simulink model "KoopmanMPC"  (R2023b)
settings: Solver=FixedStepAuto  StartTime=0.0  StopTime=inf  FixedStep=0.01  RelTol=1e-3
values from neighbouring files (symbols this model uses):
  ref_resampled_4 = [-0.0434326850921 1.00739834805 -5.2965480502 -0.0275886266971 -0.00523965410955 0.0242941259565 0.000763390489614 -0.0605545134458 1.09554308151 -5.3213592223 -0.0277571536527 -0.0053597164637 ... (2807 elements, 7x401)]    [circle_resampled_trajectory_4.mat]
undefined symbols (not defined in the file or in its folder): canChannel
libraries: canmsglib x15, canlib x11, simulink x11, dspfdesign x7, auroraNDILibrary x1
(part 1 of 2)
settings Model: Creator=86188  LastModifiedBy=86188
settings SolverCC: ConcurrentTasks=on  PositivePriorityOrder=on
settings OptimizationCC: BlockReduction=off  OptimizeBlockIOStorage=off  BufferReuse=off
settings DebuggingCC: AlgebraicLoopMsg=none  TasksWithSamePriorityMsg=none
settings HardwareCC: ProdBitPerLong=64  ProdLongLongMode=on  ProdHWDeviceType=Intel->x86-64 (Linux 64)
settings RTWCC: Description=Simulink Real-Time  SystemTargetFile=slrealtime.tlc  TemplateMakefile=slrealtime_default_tmf  Toolchain=Simulink Real-Time Toolchain  BuildConfiguration=Faster Runs  CodeExecutionProfiling=on  TargetLang=C++

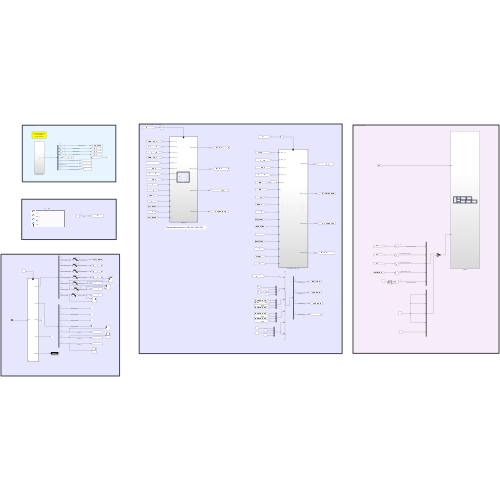
[thumbnail: Simulink's stored preview of the top-level diagram]
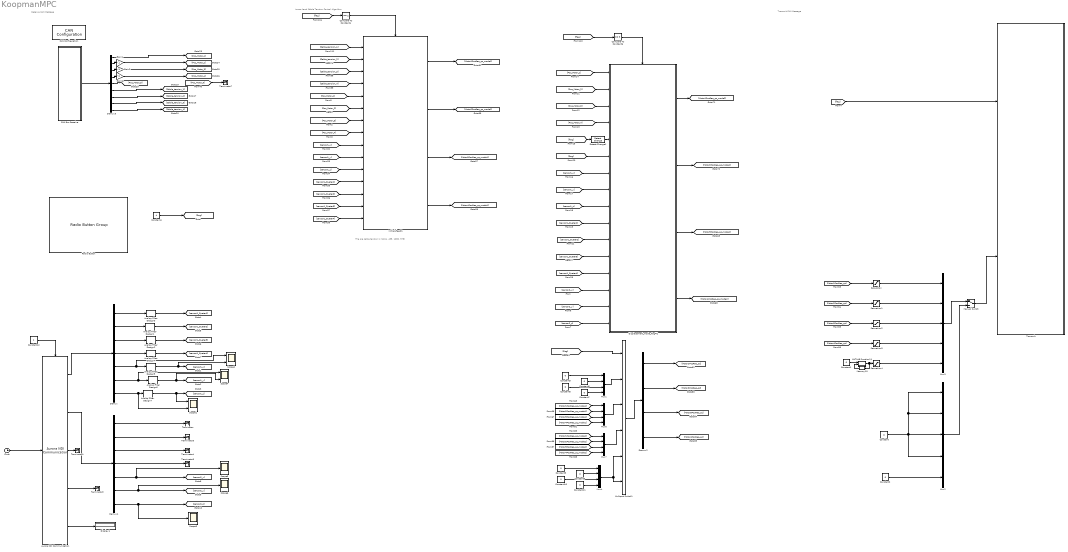
== system KoopmanMPC ==
  note: Transmit CAN Message
  note: Lower level Cable Tension Control Algorithm
  note: The pre cable tension is (1104, 455, 1080, 978)
  note: Receive CAN Message
  Analog Filter Design{1..5} (5 alike) : dspfdesign/Analog Filter Design  method=Butterworth  filttype=Lowpass  N=2  Wlo=4  Whi=80  Rp=2  Rs=40
  Analog Filter Design6 : dspfdesign/Analog Filter Design  method=Butterworth  filttype=Lowpass  N=1  Wlo=4  Whi=80  Rp=2  Rs=40
  Analog Filter Design7 : dspfdesign/Analog Filter Design  method=Butterworth  filttype=Lowpass  N=1  Wlo=4  Whi=80  Rp=2  Rs=40
  Aurora NDI Communication : auroraNDILibrary/Aurora NDI Communication  SampleFrequency=40  comNumber=4
  CAN Bus Receive : Subsystem
  CAN Configuration : canlib/CAN Configuration  BlockHandle=7005.0032  Device=PEAK-System PCAN-USB (PCAN_USBBUS1)  DeviceMenu=PEAK-System PCAN-USB (PCAN_USBBUS1)  ObjConstructor=canChannel('PEAK-System', 'PCAN_USBBUS1')  BusSpeed=500000  EnableBitParameters=off  AckMode=Normal
  Clock : Clock
  Compare To Constant4 : simulink/Logic and Bit Operations/Compare To Constant  relop===  const=2  OutDataTypeStr=boolean
  Compare To Constant6 : simulink/Logic and Bit Operations/Compare To Constant  relop===  const=3  OutDataTypeStr=boolean
  Constant{,1..3,5..11} (11 alike) : Constant  Value=0
  Constant12 : Constant
  Constant4 : Constant  Value=4
  Demux : Demux  Outputs=7
  Demux1 : Demux  Outputs=7
  Demux2 : Demux
  Demux3 : Demux  Outputs=9
  Detect Change1 : simulink/Logic and Bit Operations/Detect Change  vinit=0  OutDataTypeStr=boolean
  Displacement_mode_flag=2 : Subsystem
  Display1 : Display
  Gain1 : Gain  Gain=-1
  Gain2 : Gain  Gain=-1
  Gain6 : Gain  Gain=-1
  Initial_flag=1 : Subsystem
  MATLAB Function11 : MATLAB Function  TreatAsAtomicUnit=on
  Manual Switch : ManualSwitch
  Memory10 : Memory
  Multiport Switch1 : MultiPortSwitch  Inputs=4  DataPortForDefault=Additional data port  SaturateOnIntegerOverflow=off  InputSameDT=off
  Mux{1,4,6..7} (4 alike) : Mux
  Mux2 : Mux  Inputs=5
  Mux3 : Mux  Inputs=5
  Radio Button : RadioButtonGroup  SelectedLabel=End  ButtonGroupName=Group
      settings: Values={{'Initial', 'PreTension', 'MPC', 'End'}, [1 2 3 4]}
  Saturation{,1..3} (4 alike) : Saturate  UpperLimit=6000  LowerLimit=-6000
  Saturation4 : Saturate  UpperLimit=80  LowerLimit=-80
  Scope1 : Scope  NumInputPorts=2
  Scope2 : Scope  NumInputPorts=2
  Scope3 : Scope
  Scope4 : Scope  NumInputPorts=2
  Scope5 : Scope
  Scope6 : Scope
  Terminator{,1..5,7} (7 alike) : Terminator
  Transmit : Subsystem
  wires:
  Multiport Switch1/1 -> Demux2/1
  [Motor1PosReq_qc_mode2] -> Mux7/1
  Manual Switch/1 -> Transmit/2(Input)
  [Motor3PosReq_qc_mode2] -> Mux7/3
  [Motor2PosReq_qc_mode1] -> Mux6/2
  [Motor4PosReq_qc_mode1] -> Mux6/4
  Initial_flag=1/2(Motor2_pos_req_qc) -> [Motor2PosReq_qc_mode1]
  Initial_flag=1/3(Motor3PosReq_qc) -> [Motor3PosReq_qc_mode1]
  [flag] -> Compare To Constant4/1
  Displacement_mode_flag=2/3(Motor3PosReq_qc) -> [Motor3PosReq_qc_mode2]
  Displacement_mode_flag=2/2(Motor2_pos_req_qc) -> [Motor2PosReq_qc_mode2]
  Displacement_mode_flag=2/4(Motor4PosReq_qc) -> [Motor4PosReq_qc_mode2]
  [Motor3PosReq_qc] -> Saturation2/1
  [flag] -> Transmit/1(flag)
  [Motor1PosReq_qc_mode1] -> Mux6/1
  Displacement_mode_flag=2/1(Motor1PosReq_qc) -> [Motor1PosReq_qc_mode2]
  Initial_flag=1/4(Motor4PosReq_qc) -> [Motor4PosReq_qc_mode1]
  [Cable_tension_4] -> Initial_flag=1/4(Force_sensor_4_g)
  Compare To Constant4/1 -> Initial_flag=1/Enable
  [flag] -> Compare To Constant6/1
  [Cable_tension_3] -> Initial_flag=1/3(Force_sensor_3_g)
  [Motor3PosReq_qc_mode1] -> Mux6/3
  Mux2/1 -> Manual Switch/2
  [Motor4PosReq_qc_mode2] -> Mux7/4
  [Motor2PosReq_qc_mode2] -> Mux7/2
  Compare To Constant6/1 -> Displacement_mode_flag=2/Enable
  [Cable_tension_2] -> Initial_flag=1/2(Force_sensor_2_g)
  [Cable_tension_1] -> Initial_flag=1/1(Force_sensor_1_g)
  Initial_flag=1/1(Motor1PosReq_qc) -> [Motor1PosReq_qc_mode1]
  [Pos_Motor_2] -> Displacement_mode_flag=2/2(Pos_Motor_2_qc)
  [Pos_Motor_1] -> Displacement_mode_flag=2/1(Pos_Motor_1_qc)
  [Pos_Motor_3] -> Displacement_mode_flag=2/3(Pos_Motor_3_qc)
  [Pos_Motor_4] -> Displacement_mode_flag=2/4(Pos_Motor_4_qc)
  [flag] -> Detect Change1/1
  [flag] -> Displacement_mode_flag=2/6(flag)
  Detect Change1/1 -> Displacement_mode_flag=2/5(flag_change)
  Saturation4/1 -> Mux3/5  "Motor5PosReq_qc_final"
  Mux3/1 -> Manual Switch/1
  Saturation3/1 -> Mux3/4  "Motor4PosReq_qc_final"
  Saturation/1 -> Mux3/1  "Motor1PosReq_qc_final"
  Saturation1/1 -> Mux3/2  "Motor2PosReq_qc_final"
  Saturation2/1 -> Mux3/3  "Motor3PosReq_qc_final"
  [Motor2PosReq_qc] -> Saturation1/1
  [Motor4PosReq_qc] -> Saturation3/1
  MATLAB Function11/1(y) -> Memory10/1, Saturation4/1
  Memory10/1 -> MATLAB Function11/2(u_last)
  Demux2/1 -> [Motor1PosReq_qc]  "Motor1PosReq_qc"
  Demux2/2 -> [Motor2PosReq_qc]  "Motor2PosReq_qc"
  Demux2/3 -> [Motor3PosReq_qc]  "Motor3PosReq_qc"
  Demux2/4 -> [Motor4PosReq_qc]  "Motor4PosReq_qc"
  Constant1/1 -> MATLAB Function11/1(u)
  Constant/1 -> Mux2/4, Mux2/1, Mux2/2, Mux2/3
  Constant2/1 -> Mux2/5
  [Pos_Motor_1] -> Initial_flag=1/5(Pos_Motor_1_qc)
  [Pos_Motor_2] -> Initial_flag=1/6(Pos_Motor_2_qc)
  [Pos_Motor_3] -> Initial_flag=1/7(Pos_Motor_3_qc)
  [Pos_Motor_4] -> Initial_flag=1/8(Pos_Motor_4_qc)
  [flag] -> Multiport Switch1/1
  [Motor1PosReq_qc] -> Saturation/1
  [sensor1_Quater1] -> Displacement_mode_flag=2/10(q0)
  [sensor1_z] -> Displacement_mode_flag=2/9(z)
  [sensor1_Quater2] -> Displacement_mode_flag=2/11(q1)
  [sensor1_y] -> Displacement_mode_flag=2/8(y)
  [sensor1_Quater3] -> Displacement_mode_flag=2/12(q2)
  [sensor1_x] -> Displacement_mode_flag=2/7(x)
  [sensor1_Quater4] -> Displacement_mode_flag=2/13(q3)
  [sensor1_x] -> Initial_flag=1/9(x)
  [sensor1_y] -> Initial_flag=1/10(y)
  [sensor1_z] -> Initial_flag=1/11(z)
  [sensor1_Quater1] -> Initial_flag=1/12(q0)
  [sensor1_Quater2] -> Initial_flag=1/13(q1)
  [sensor1_Quater3] -> Initial_flag=1/14(q2)
  [sensor1_Quater4] -> Initial_flag=1/15(q3)
  [Pos_Motor_5] -> Terminator7/1
  Gain1/1 -> [Pos_Motor_2]  "RealPos_Motor_2"
  Demux3/2 -> Gain1/1
  Demux3/4 -> Gain6/1
  Gain6/1 -> [Pos_Motor_4]  "RealPos_Motor_4"
  Demux3/7 -> [Cable_tension_2]  "force_sensor_2_org"
  Gain2/1 -> [Pos_Motor_3]  "RealPos_Motor_3"
  Demux3/8 -> [Cable_tension_3]  "force_sensor_3_org"
  Demux3/5 -> [Pos_Motor_5]
  Demux3/3 -> Gain2/1
  Demux3/1 -> [Pos_Motor_1]  "RealPos_Motor_1"
  Demux3/6 -> [Cable_tension_1]  "force_sensor_1_org"
  CAN Bus Receive/1(Outport) -> Demux3/1
  Demux3/9 -> [Cable_tension_4]  "force_sensor_4_org"
  Mux6/1 -> Multiport Switch1/3
  Mux7/1 -> Multiport Switch1/4
  Constant7/1 -> Mux1/4
  Constant5/1 -> Mux1/2
  Constant6/1 -> Mux1/3
  Mux1/1 -> Multiport Switch1/2
  Constant3/1 -> Mux1/1
  Constant4/1 -> [flag]  "flag"
  Constant10/1 -> Mux4/3
  Constant9/1 -> Mux4/2
  Constant11/1 -> Mux4/4
  Mux4/1 -> Multiport Switch1/6, Multiport Switch1/5
  Constant8/1 -> Mux4/1
  Demux1/2 -> Terminator3/1  "sensor2_Quater2"
  Demux1/6 -> Scope6/1, [sensor2_y]  "sensor2_y"
  Demux1/4 -> Terminator5/1  "sensor2_Quater4"
  Aurora NDI Communication/2 -> Demux1/1
  Analog Filter Design5/1 -> Scope2/2, [sensor1_x]  "sensor1_x_after"
  Demux1/1 -> Terminator/1  "sensor2_Quater1"
  Aurora NDI Communication/5 -> Display1/1
  Demux/7 -> Analog Filter Design7/1, Scope1/2  "sensor1_z_before"
  Analog Filter Design7/1 -> Scope1/1, [sensor1_z]  "sensor1_z_after"
  Demux1/5 -> [sensor2_x], Scope5/1  "sensor2_x"
  Analog Filter Design6/1 -> Scope4/2, [sensor1_y]  "sensor1_y_after"
  Demux/4 -> Analog Filter Design4/1  "sensor1_Quater4_before"
  Demux1/3 -> Terminator4/1  "sensor2_Quater3"
  Analog Filter Design4/1 -> [sensor1_Quater4]  "sensor1_Quater4_after"
  Demux/5 -> Scope2/1, Analog Filter Design5/1  "sensor1_x_before"
  Analog Filter Design2/1 -> [sensor1_Quater3]  "sensor1_Quater3_after"
  Demux1/7 -> Scope3/1, [sensor2_z]  "sensor2_z"
  Demux/6 -> Analog Filter Design6/1, Scope4/1  "sensor1_y_before"
  Analog Filter Design3/1 -> [sensor1_Quater1]  "sensor1_Quater1_after"
  Demux/1 -> Analog Filter Design3/1  "sensor1_Quater1_before"
  Aurora NDI Communication/1 -> Demux/1
  Demux/2 -> Analog Filter Design1/1  "sensor1_Quater2_before"
  Constant12/1 -> Aurora NDI Communication/Enable
  Aurora NDI Communication/3 -> Terminator1/1
  Clock/1 -> Aurora NDI Communication/1
  Aurora NDI Communication/4 -> Terminator2/1
  Analog Filter Design1/1 -> [sensor1_Quater2]  "sensor1_Quater2_after"
  Demux/3 -> Analog Filter Design2/1  "sensor1_Quater3_before"
  [sensor2_x] -> Displacement_mode_flag=2/14(x1)
  [sensor2_z] -> Displacement_mode_flag=2/16(z1)
  [sensor2_y] -> Displacement_mode_flag=2/15(y1)

== system KoopmanMPC/CAN Bus Receive ==
  CAN Receive : canlib/CAN Receive  BlockHandle=1206.0054  Device=PEAK-System PCAN-USB (PCAN_USBBUS1)  DeviceMenu=PEAK-System PCAN-USB (PCAN_USBBUS1)  ObjConstructor=canChannel('PEAK-System', 'PCAN_USBBUS1')  EnableStandardIDsFilter=off  StdIDsCombo=Allow all  StandardIDs=0  EnableExtendedIDsFilter=off  ExtIDsCombo=Allow all  ExtendedIDs=0  SampleTime=0.01  MsgsPerTimestep=all  InternalFilterUpdateStatus=on  BusOutput=on
  Rate Transition : RateTransition  OutPortSampleTime=0.01
  Subsystem : Subsystem
  Outport : Outport
  wires:
  CAN Receive/1 -> Subsystem/Trigger
  Subsystem/1(Outport1) -> Rate Transition/1
  Rate Transition/1 -> Outport/1
  CAN Receive/2 -> Subsystem/1(In2)

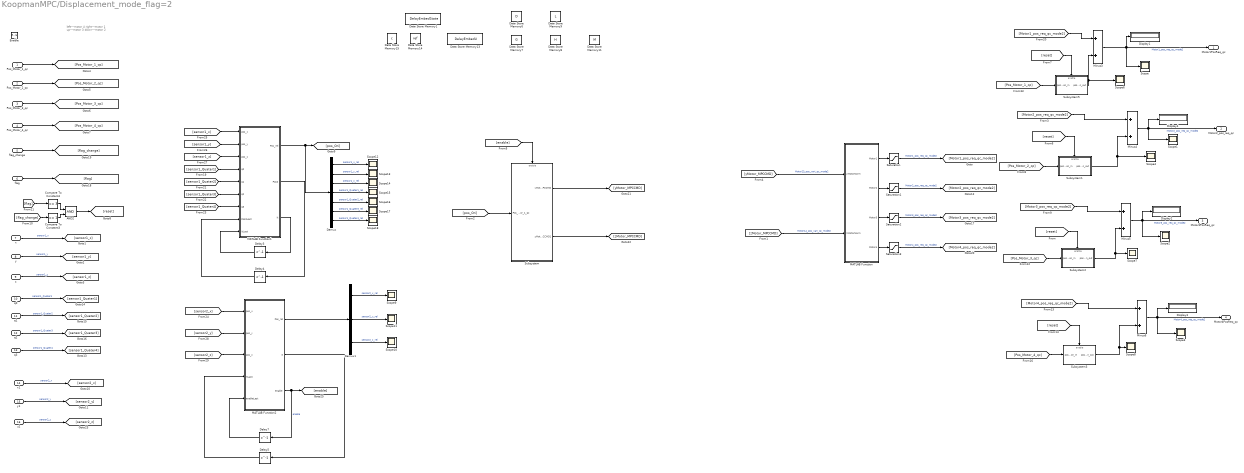
== system KoopmanMPC/Displacement_mode_flag=2 ==
  note: left---motor 4
      | right---motor 1
      | up---motor 3
      | down---motor 2
  Pos_Motor_1_qc : Inport
  Pos_Motor_2_qc : Inport  Port=2
  Pos_Motor_3_qc : Inport  Port=3
  Pos_Motor_4_qc : Inport  Port=4
  flag_change : Inport  Port=5
  flag : Inport  Port=6
  x : Inport  Port=7
  y : Inport  Port=8
  z : Inport  Port=9
  q0 : Inport  Port=10
  q1 : Inport  Port=11
  q2 : Inport  Port=12
  q3 : Inport  Port=13
  x1 : Inport  Port=14
  y1 : Inport  Port=15
  z1 : Inport  Port=16
  Enable : EnablePort  StatesWhenEnabling=reset
  AND2 : Logic  IconShape=distinctive  AllPortsSameDT=off  OutDataTypeStr=boolean
  Compare To Constant3 : simulink/Logic and Bit Operations/Compare To Constant  relop===  const=1  OutDataTypeStr=boolean
  Compare To Constant4 : simulink/Logic and Bit Operations/Compare To Constant  relop===  const=3  OutDataTypeStr=boolean
  Data Store Memory1 : DataStoreMemory  DataStoreName=DelayEmbedState  WriteAfterWriteMsg=warning  InitialValue=zeros(7,2)  ShowAdditionalParam=off  OutDataTypeStr=double
  Data Store Memory11 : DataStoreMemory  DataStoreName=M  WriteAfterWriteMsg=warning  InitialValue=M  ShowAdditionalParam=off  OutDataTypeStr=double
  Data Store Memory13 : DataStoreMemory  DataStoreName=DelayEmbedU  WriteAfterWriteMsg=warning  InitialValue=zeros(2,2)  ShowAdditionalParam=off  OutDataTypeStr=double
  Data Store Memory14 : DataStoreMemory  DataStoreName=ref  WriteAfterWriteMsg=warning  InitialValue=[ref_resampled_4,ref_resampled_4]  ShowAdditionalParam=off  OutDataTypeStr=double
  Data Store Memory15 : DataStoreMemory  DataStoreName=c  WriteAfterWriteMsg=warning  InitialValue=c  ShowAdditionalParam=off  OutDataTypeStr=double
  Data Store Memory6 : DataStoreMemory  DataStoreName=D  WriteAfterWriteMsg=warning  InitialValue=D  ShowAdditionalParam=off  OutDataTypeStr=double
  Data Store Memory7 : DataStoreMemory  DataStoreName=G  WriteAfterWriteMsg=warning  InitialValue=G  ShowAdditionalParam=off  OutDataTypeStr=double
  Data Store Memory8 : DataStoreMemory  DataStoreName=H  WriteAfterWriteMsg=warning  InitialValue=H  ShowAdditionalParam=off  OutDataTypeStr=double
  Data Store Memory9 : DataStoreMemory  DataStoreName=L  WriteAfterWriteMsg=warning  InitialValue=L  ShowAdditionalParam=off  OutDataTypeStr=double
  Delay3 : Delay  DelayLength=1  InitialCondition=1
  Delay4 : Delay  DelayLength=1  InitialCondition=ones(1,7)
  Delay5 : Delay  DelayLength=1  InitialCondition=1
  Delay7 : Delay  DelayLength=1  InitialCondition=0
  Demux : Demux  Outputs=7
  Demux1 : Demux  Outputs=3
  Display{1..4} (4 alike) : Display
  MATLAB Function : MATLAB Function  TreatAsAtomicUnit=on
  MATLAB Function1 : MATLAB Function  TreatAsAtomicUnit=on
  MATLAB Function2 : MATLAB Function  TreatAsAtomicUnit=on
  Minus{3..6} (4 alike) : Sum
  Saturation{,1..3} (4 alike) : Saturate  UpperLimit=1200  LowerLimit=-1200
  Scope{,1..4,6..18} (18 alike) : Scope
  Subsystem : Subsystem
  Subsystem1 : Subsystem
  Subsystem2 : Subsystem
  Subsystem3 : Subsystem
  Subsystem5 : Subsystem
  Motor1PosReq_qc : Outport
  Motor2_pos_req_qc : Outport  Port=2
  Motor3PosReq_qc : Outport  Port=3
  Motor4PosReq_qc : Outport  Port=4
  wires:
  Pos_Motor_4_qc/1 -> [Pos_Motor_4_qc]
  Pos_Motor_3_qc/1 -> [Pos_Motor_3_qc]
  Pos_Motor_2_qc/1 -> [Pos_Motor_2_qc]
  Pos_Motor_1_qc/1 -> [Pos_Motor_1_qc]
  flag/1 -> [flag]
  flag_change/1 -> [flag_change]
  [Pos_Motor_1_qc] -> Subsystem5/1(position_in)
  [reset] -> Subsystem5/Enable
  [Motor1_pos_req_qc_mode2] -> Minus3/1
  Minus3/1 -> Scope/1, Display1/1, Motor1PosReq_qc/1  "Motor1_pos_req_qc_mode2"
  Subsystem5/1(position_out) -> Minus3/2, Scope6/1
  [Motor2_pos_req_qc_mode2] -> Minus4/1
  [reset] -> Subsystem1/Enable
  [Pos_Motor_2_qc] -> Subsystem1/1(position_in)
  Minus4/1 -> Scope1/1, Display4/1, Motor2_pos_req_qc/1  "Motor2_pos_req_qc_mode2"
  Minus5/1 -> Scope2/1, Motor3PosReq_qc/1, Display2/1  "Motor3_pos_req_qc_mode2"
  [reset] -> Subsystem2/Enable
  [Pos_Motor_3_qc] -> Subsystem2/1(position_in)
  [Motor3_pos_req_qc_mode2] -> Minus5/1
  Minus6/1 -> Scope3/1, Motor4PosReq_qc/1, Display3/1  "Motor4_pos_req_qc_mode2"
  [reset] -> Subsystem3/Enable
  [Pos_Motor_4_qc] -> Subsystem3/1(position_in)
  [Motor4_pos_req_qc_mode2] -> Minus6/1
  Compare To Constant4/1 -> AND2/1
  Compare To Constant3/1 -> AND2/2
  [flag_change] -> Compare To Constant3/1
  [flag] -> Compare To Constant4/1
  AND2/1 -> [reset]
  Subsystem2/1(position_out) -> Minus5/2, Scope7/1
  Subsystem3/1(position_out) -> Minus6/2, Scope8/1
  Subsystem1/1(position_out) -> Minus4/2, Scope4/1
  x/1 -> [sensor1_x]  "sensor1_x"
  y/1 -> [sensor1_y]  "sensor1_y"
  z/1 -> [sensor1_z]  "sensor1_z"
  q0/1 -> [sensor1_Quater1]  "sensor1_Quater1"
  q1/1 -> [sensor1_Quater2]  "sensor1_Quater2"
  q3/1 -> [sensor1_Quater4]  "sensor1_Quater4"
  q2/1 -> [sensor1_Quater3]  "sensor1_Quater3"
  Demux/2 -> Scope13/1  "sensor1_y_rel"
  Demux/7 -> Scope18/1  "sensor1_Quater4_rel"
  [sensor1_Quater1] -> MATLAB Function1/4(q0)
  Demux/1 -> Scope12/1  "sensor1_x_rel"
  [sensor1_Quater3] -> MATLAB Function1/6(q2)
  Demux/3 -> Scope14/1  "sensor1_z_rel"
  Demux/6 -> Scope17/1  "sensor1_Quater3_rel"
  Demux/4 -> Scope15/1  "sensor1_Quater1_rel"
  Delay4/1 -> MATLAB Function1/8(Pos0Last)
  Delay3/1 -> MATLAB Function1/9(itLast)
  [sensor1_Quater2] -> MATLAB Function1/5(q1)
  MATLAB Function1/2(Pos0) -> Delay4/1
  MATLAB Function1/1(Pos_rel) -> Demux/1, [pos_Ori]
  [sensor1_z] -> MATLAB Function1/3(pos_z)
  [sensor1_y] -> MATLAB Function1/2(pos_y)
  [sensor1_x] -> MATLAB Function1/1(pos_x)
  MATLAB Function1/3(it) -> Delay3/1
  Demux/5 -> Scope16/1  "sensor1_Quater2_rel"
  [sensor1_Quater4] -> MATLAB Function1/7(q3)
  Saturation2/1 -> [Motor3_pos_req_qc_mode2]  "Motor3_pos_req_qc_mode2"
  Saturation3/1 -> [Motor4_pos_req_qc_mode2]  "Motor4_pos_req_qc_mode2"
  MATLAB Function/3(Motor3) -> Saturation2/1
  MATLAB Function/1(Motor1) -> Saturation/1
  MATLAB Function/4(Motor4) -> Saturation3/1
  Saturation1/1 -> [Motor2_pos_req_qc_mode2]  "Motor2_pos_req_qc_mode2"
  Saturation/1 -> [Motor1_pos_req_qc_mode2]  "Motor1_pos_req_qc_mode2"
  MATLAB Function/2(Motor2) -> Saturation1/1
  [yMotor_MPCCMD] -> MATLAB Function/1(yMotorNorm)  "Motor23_pos_vari_qc_mode2"
  [zMotor_MPCCMD] -> MATLAB Function/2(zMotorNorm)  "Motor14_pos_vari_qc_mode2"
  Delay5/1 -> MATLAB Function2/4(itLast)
  MATLAB Function2/3(enable) -> Delay7/1, [enable]  "enable"
  Delay7/1 -> MATLAB Function2/5(enableLast)
  [sensor2_y] -> MATLAB Function2/2(pos_y)
  Demux1/2 -> Scope11/1  "sensor2_y_rel"
  [sensor2_x] -> MATLAB Function2/1(pos_x)
  Demux1/3 -> Scope10/1  "sensor2_z_rel"
  Demux1/1 -> Scope9/1  "sensor2_x_rel"
  [sensor2_z] -> MATLAB Function2/3(pos_z)
  MATLAB Function2/1(Pos_rel) -> Demux1/1
  MATLAB Function2/2(it) -> Delay5/1
  y1/1 -> [sensor2_y]  "sensor2_y"
  z1/1 -> [sensor2_z]  "sensor2_z"
  x1/1 -> [sensor2_x]  "sensor2_x"
  [pos_Ori] -> Subsystem/1(Pos_Motor_1_qc)
  [enable] -> Subsystem/Enable
  Subsystem/1(yMotor_MPCCMD) -> [yMotor_MPCCMD]
  Subsystem/2(zMotor_MPCCMD1) -> [zMotor_MPCCMD]

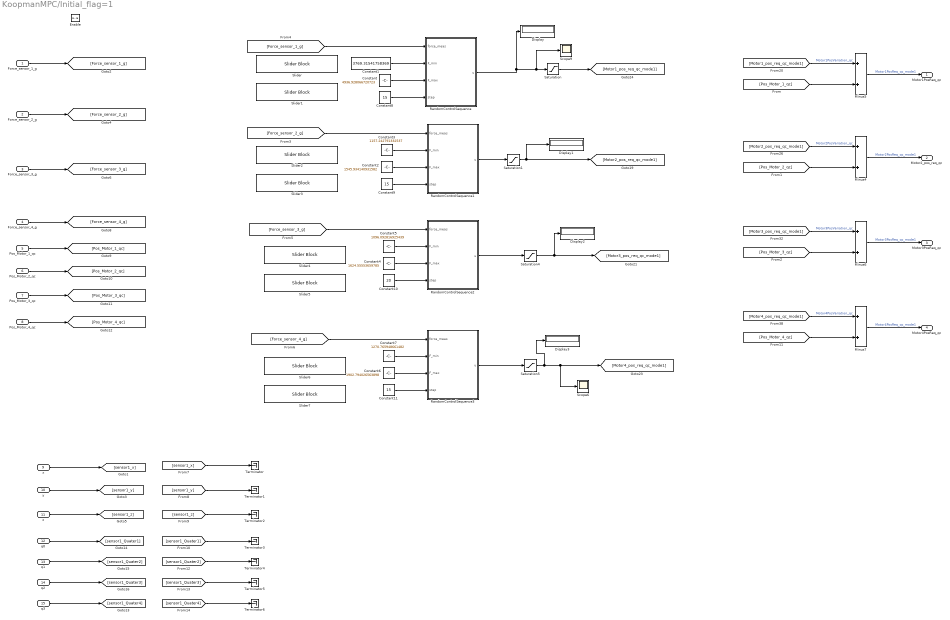
== system KoopmanMPC/Initial_flag=1 ==
  Force_sensor_1_g : Inport
  Force_sensor_2_g : Inport  Port=2
  Force_sensor_3_g : Inport  Port=3
  Force_sensor_4_g : Inport  Port=4
  Pos_Motor_1_qc : Inport  Port=5
  Pos_Motor_2_qc : Inport  Port=6
  Pos_Motor_3_qc : Inport  Port=7
  Pos_Motor_4_qc : Inport  Port=8
  x : Inport  Port=9
  y : Inport  Port=10
  z : Inport  Port=11
  q0 : Inport  Port=12
  q1 : Inport  Port=13
  q2 : Inport  Port=14
  q3 : Inport  Port=15
  Enable : EnablePort
  Constant : Constant  Value=4936.928066720723
  Constant1 : Constant  Value=3769.31541758369
  Constant10 : Constant  Value=20
  Constant11 : Constant  Value=15
  Constant2 : Constant  Value=1545.934140931582
  Constant3 : Constant  Value=1157.242791332537
  Constant4 : Constant  Value=1624.55553659785
  Constant5 : Constant  Value=1096.092816925439
  Constant6 : Constant  Value=1902.794026563898
  Constant7 : Constant  Value=1270.765948661482
  Constant8 : Constant  Value=15
  Constant9 : Constant  Value=15
  Display{,1..3} (4 alike) : Display
  Minus{4..7} (4 alike) : Sum
  RandomControlSequence : MATLAB Function  TreatAsAtomicUnit=on
  RandomControlSequence1 : MATLAB Function  TreatAsAtomicUnit=on
  RandomControlSequence2 : MATLAB Function  TreatAsAtomicUnit=on
  RandomControlSequence3 : MATLAB Function  TreatAsAtomicUnit=on
  Saturation{,1,4..5} (4 alike) : Saturate  UpperLimit=200  LowerLimit=-200
  Scope6 : Scope
  Scope9 : Scope
  Slider : SliderBlock  ScaleMin=500  ScaleMax=4000
  Slider1 : SliderBlock  ScaleMin=500  ScaleMax=5000
  Slider2 : SliderBlock  ScaleMin=1000  ScaleMax=3000
  Slider3 : SliderBlock  ScaleMin=1200  ScaleMax=3000
  Slider4 : SliderBlock  ScaleMin=1000  ScaleMax=3000
  Slider5 : SliderBlock  ScaleMin=1200  ScaleMax=3000
  Slider6 : SliderBlock  ScaleMin=500  ScaleMax=4000
  Slider7 : SliderBlock  ScaleMin=500  ScaleMax=4000
  Terminator{,1..6} (7 alike) : Terminator
  Motor1PosReq_qc : Outport
  Motor2_pos_req_qc : Outport  Port=2
  Motor3PosReq_qc : Outport  Port=3
  Motor4PosReq_qc : Outport  Port=4
  wires:
  [Force_sensor_1_g] -> RandomControlSequence/1(force_meas)
  [Force_sensor_4_g] -> RandomControlSequence3/1(force_meas)
  Saturation/1 -> [Motor1_pos_req_qc_mode1]
  [Force_sensor_3_g] -> RandomControlSequence2/1(force_meas)
  RandomControlSequence/1(u) -> Display/1, Scope9/1, Saturation/1
  Saturation4/1 -> Display2/1, [Motor3_pos_req_qc_mode1]
  Force_sensor_3_g/1 -> [Force_sensor_3_g]
  Force_sensor_4_g/1 -> [Force_sensor_4_g]
  Force_sensor_2_g/1 -> [Force_sensor_2_g]
  Force_sensor_1_g/1 -> [Force_sensor_1_g]
  Saturation1/1 -> [Motor2_pos_req_qc_mode1], Display1/1
  Saturation5/1 -> Display3/1, Scope6/1, [Motor4_pos_req_qc_mode1]
  Pos_Motor_4_qc/1 -> [Pos_Motor_4_qc]
  Pos_Motor_1_qc/1 -> [Pos_Motor_1_qc]
  Pos_Motor_3_qc/1 -> [Pos_Motor_3_qc]
  Pos_Motor_2_qc/1 -> [Pos_Motor_2_qc]
  Minus5/1 -> Motor1PosReq_qc/1  "Motor1PosReq_qc_mode1"
  [Motor1_pos_req_qc_mode1] -> Minus5/1  "Motor1PosVariation_qc"
  [Pos_Motor_1_qc] -> Minus5/2
  Minus4/1 -> Motor2_pos_req_qc/1  "Motor2PosReq_qc_mode1"
  [Motor2_pos_req_qc_mode1] -> Minus4/1  "Motor2PosVariation_qc"
  [Pos_Motor_2_qc] -> Minus4/2
  [Motor3_pos_req_qc_mode1] -> Minus6/1  "Motor3PosVariation_qc"
  Minus6/1 -> Motor3PosReq_qc/1  "Motor3PosReq_qc_mode1"
  [Pos_Motor_3_qc] -> Minus6/2
  [Motor4_pos_req_qc_mode1] -> Minus7/1  "Motor4PosVariation_qc"
  Minus7/1 -> Motor4PosReq_qc/1  "Motor4PosReq_qc_mode1"
  [Pos_Motor_4_qc] -> Minus7/2
  Constant/1 -> RandomControlSequence/3(F_max)
  Constant1/1 -> RandomControlSequence/2(F_min)
  RandomControlSequence1/1(u) -> Saturation1/1
  [Force_sensor_2_g] -> RandomControlSequence1/1(force_meas)
  Constant3/1 -> RandomControlSequence1/2(F_min)
  Constant2/1 -> RandomControlSequence1/3(F_max)
  RandomControlSequence2/1(u) -> Saturation4/1
  Constant4/1 -> RandomControlSequence2/3(F_max)
  Constant5/1 -> RandomControlSequence2/2(F_min)
  RandomControlSequence3/1(u) -> Saturation5/1
  Constant7/1 -> RandomControlSequence3/2(F_min)
  Constant6/1 -> RandomControlSequence3/3(F_max)
  Constant8/1 -> RandomControlSequence/4(step)
  Constant9/1 -> RandomControlSequence1/4(step)
  Constant10/1 -> RandomControlSequence2/4(step)
  Constant11/1 -> RandomControlSequence3/4(step)
  z/1 -> [sensor1_z]
  x/1 -> [sensor1_x]
  y/1 -> [sensor1_y]
  q3/1 -> [sensor1_Quater4]
  q2/1 -> [sensor1_Quater3]
  q1/1 -> [sensor1_Quater2]
  q0/1 -> [sensor1_Quater1]
  [sensor1_x] -> Terminator/1
  [sensor1_y] -> Terminator1/1
  [sensor1_z] -> Terminator2/1
  [sensor1_Quater1] -> Terminator3/1
  [sensor1_Quater2] -> Terminator4/1
  [sensor1_Quater3] -> Terminator5/1
  [sensor1_Quater4] -> Terminator6/1

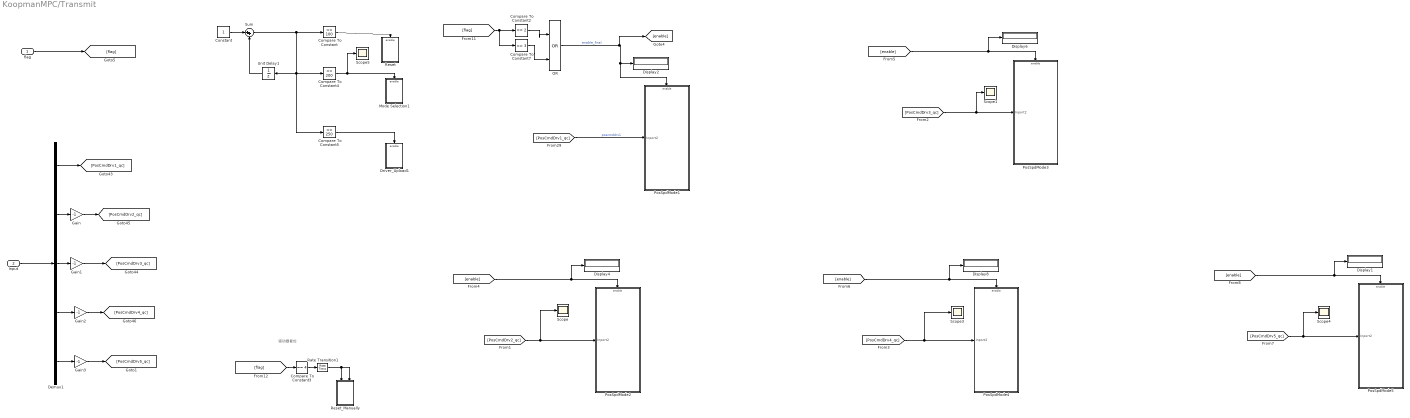
== system KoopmanMPC/Transmit ==
  note: 驱动器复位
  flag : Inport
  Input : Inport  Port=2
  Compare To Constant : simulink/Logic and Bit Operations/Compare To Constant  relop===  const=100  OutDataTypeStr=boolean
  Compare To Constant2 : simulink/Logic and Bit Operations/Compare To Constant  relop===  const=2  OutDataTypeStr=boolean
  Compare To Constant3 : simulink/Logic and Bit Operations/Compare To Constant  relop===  const=4  OutDataTypeStr=boolean
  Compare To Constant4 : simulink/Logic and Bit Operations/Compare To Constant  relop===  const=200  OutDataTypeStr=boolean
  Compare To Constant5 : simulink/Logic and Bit Operations/Compare To Constant  relop===  const=250  OutDataTypeStr=boolean
  Compare To Constant7 : simulink/Logic and Bit Operations/Compare To Constant  relop===  const=3  OutDataTypeStr=boolean
  Constant : Constant
  Demux1 : Demux  Outputs=5
  Display{1..2,4,6,8} (5 alike) : Display
  Driver_Upload1 : Subsystem
  Gain{,1..3} (4 alike) : Gain  Gain=-1
  Mode Selection1 : Subsystem  ScheduleAs=Aperiodic partition  PartitionName=TEMP_PRECOMP_PARTITION_NAME_MessageTriggeredSubsystem
  OR : Logic  Operator=OR  IconShape=distinctive  AllPortsSameDT=off  OutDataTypeStr=boolean
  PosSpdMode1 : Subsystem
  PosSpdMode2 : Subsystem
  PosSpdMode3 : Subsystem
  PosSpdMode4 : Subsystem
  PosSpdMode5 : Subsystem
  Rate Transition1 : RateTransition  OutPortSampleTime=1
  Reset : Subsystem
  Reset_Manually : Subsystem
  Scope{,1,3..5} (5 alike) : Scope
  Sum : Sum  Inputs=|++  InputSameDT=on  SaturateOnIntegerOverflow=on  OutDataTypeStr=Inherit: Same as first input
  Unit Delay1 : UnitDelay  SampleTime=-1  HasFrameUpgradeWarning=on
  wires:
  OR/1 -> [enable], PosSpdMode1/Enable, Display2/1  "enable_final"
  [flag] -> Compare To Constant3/1
  Compare To Constant3/1 -> Rate Transition1/1
  Rate Transition1/1 -> Reset_Manually/Trigger, Reset_Manually/Enable
  Demux1/1 -> [PosCmdDrv1_qc]
  Demux1/3 -> Gain1/1
  Demux1/4 -> Gain2/1
  Input/1 -> Demux1/1
  Demux1/2 -> Gain/1
  [enable] -> Display4/1, PosSpdMode2/Enable
  [enable] -> Display6/1, PosSpdMode3/Enable
  [enable] -> Display8/1, PosSpdMode4/Enable
  Gain/1 -> [PosCmdDrv2_qc]
  Gain1/1 -> [PosCmdDrv3_qc]
  Gain2/1 -> [PosCmdDrv4_qc]
  [PosCmdDrv1_qc] -> PosSpdMode1/1(Inport2)  "poscmddrv1"
  [PosCmdDrv3_qc] -> Scope1/1, PosSpdMode3/1(Inport2)
  [PosCmdDrv2_qc] -> Scope/1, PosSpdMode2/1(Inport2)
  [PosCmdDrv4_qc] -> Scope3/1, PosSpdMode4/1(Inport2)
  [enable] -> Display1/1, PosSpdMode5/Enable
  [PosCmdDrv5_qc] -> Scope4/1, PosSpdMode5/1(Inport2)
  Demux1/5 -> Gain3/1
  Gain3/1 -> [PosCmdDrv5_qc]
  flag/1 -> [flag]
  [flag] -> Compare To Constant7/1, Compare To Constant2/1
  Compare To Constant2/1 -> OR/1
  Compare To Constant7/1 -> OR/2
  Compare To Constant4/1 -> Scope5/1, Mode Selection1/Enable
  Compare To Constant/1 -> Reset/Enable
  Compare To Constant5/1 -> Driver_Upload1/Enable
  Sum/1 -> Compare To Constant5/1, Compare To Constant4/1, Unit Delay1/1, Compare To Constant/1
  Unit Delay1/1 -> Sum/2
  Constant/1 -> Sum/1

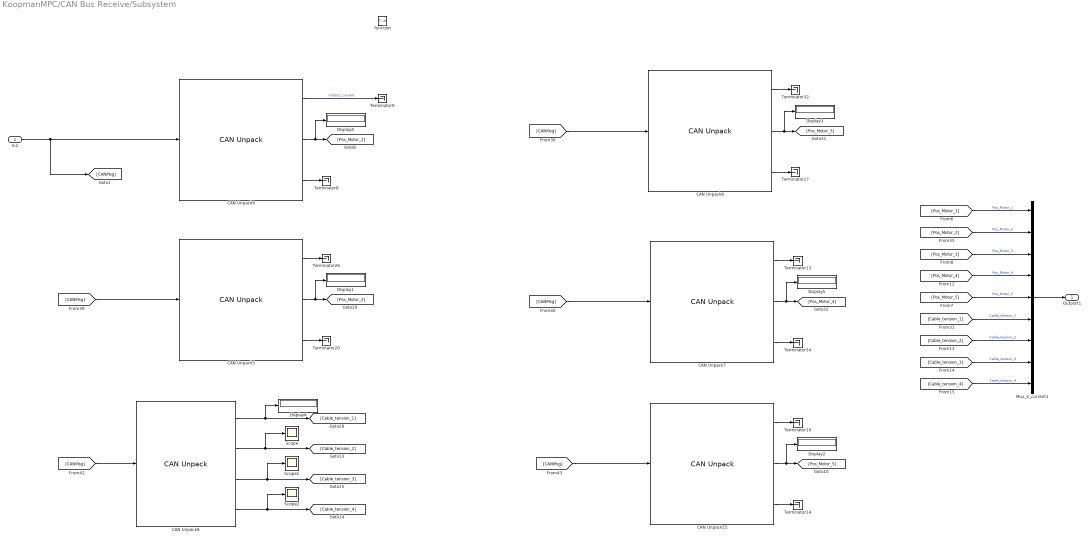
== system KoopmanMPC/CAN Bus Receive/Subsystem ==
  In2 : Inport
  function : TriggerPort  TriggerType=function-call  VariantControl=Variant
  CAN Unpack15 : canmsglib/CAN Unpack  CANdbFile=E:\OneDrive\OneDrive - The Chinese University of Hong Kong\文档\Research\SRIL\12nd\Experiment\Simulink\RoboModule0729.dbc  MsgList=Feedback_curvelpos_Dr5  MsgName=Feedback_curvelpos_Dr5  MsgIDType=Standard (11-bit identifier)  MsgIdentifier=91  MsgLength=8  SignalInfo={'real_current','8','16','BE','signed','Standard','0','1','0','-Inf','Inf';'real_position','56','32','BE','signed','Standard','0','1','0','-Inf','Inf';'real_velocity','24','16','BE','signed','Standard','0','1','0','-Inf','Inf'}  IDPort=off  TimestampPort=off  ErrorPort=off  RemotePort=off  LengthPort=off  StatusPort=off  ApplyMinMax=off
      settings: DataFormat=CANdb specified signals
  CAN Unpack5 : canmsglib/CAN Unpack  CANdbFile=E:\OneDrive\OneDrive - The Chinese University of Hong Kong\文档\Research\SRIL\12nd\Experiment\Simulink\RoboModule0729.dbc  MsgList=Feedback_curvelpos_Dv2  MsgName=Feedback_curvelpos_Dv2  MsgIDType=Standard (11-bit identifier)  MsgIdentifier=43  MsgLength=8  SignalInfo={'real_current','8','16','BE','signed','Standard','0','1','0','-Inf','Inf';'real_position','56','32','BE','signed','Standard','0','1','0','-Inf','Inf';'real_velocity','24','16','BE','signed','Standard','0','1','0','-Inf','Inf'}  IDPort=off  TimestampPort=off  ErrorPort=off  RemotePort=off  LengthPort=off  StatusPort=off  ApplyMinMax=off
      settings: DataFormat=CANdb specified signals
  CAN Unpack6 : canmsglib/CAN Unpack  CANdbFile=E:\OneDrive\OneDrive - The Chinese University of Hong Kong\文档\Research\SRIL\12nd\Experiment\Simulink\RoboModule0729.dbc  MsgList=Feedback_curvelpos_Dv3  MsgName=Feedback_curvelpos_Dv3  MsgIDType=Standard (11-bit identifier)  MsgIdentifier=59  MsgLength=8  SignalInfo={'real_current','8','16','BE','signed','Standard','0','1','0','-Inf','Inf';'real_position','56','32','BE','signed','Standard','0','1','0','-Inf','Inf';'real_velocity','24','16','BE','signed','Standard','0','1','0','-Inf','Inf'}  IDPort=off  TimestampPort=off  ErrorPort=off  RemotePort=off  LengthPort=off  StatusPort=off  ApplyMinMax=off
      settings: DataFormat=CANdb specified signals
  CAN Unpack7 : canmsglib/CAN Unpack  CANdbFile=E:\OneDrive\OneDrive - The Chinese University of Hong Kong\文档\Research\SRIL\12nd\Experiment\Simulink\RoboModule0729.dbc  MsgList=Feedback_curvelpos_Dr4  MsgName=Feedback_curvelpos_Dr4  MsgIDType=Standard (11-bit identifier)  MsgIdentifier=75  MsgLength=8  SignalInfo={'real_current','8','16','BE','signed','Standard','0','1','0','-Inf','Inf';'real_position','56','32','BE','signed','Standard','0','1','0','-Inf','Inf';'real_velocity','24','16','BE','signed','Standard','0','1','0','-Inf','Inf'}  IDPort=off  TimestampPort=off  ErrorPort=off  RemotePort=off  LengthPort=off  StatusPort=off  ApplyMinMax=off
      settings: DataFormat=CANdb specified signals
  CAN Unpack8 : canmsglib/CAN Unpack  CANdbFile=E:\OneDrive\OneDrive - The Chinese University of Hong Kong\文档\Research\SRIL\12nd\Experiment\Simulink\RoboModule0729.dbc  MsgList=Cable_tension  MsgName=Cable_tension  MsgIDType=Extended (29-bit identifier)  MsgIdentifier=529024  MsgLength=8  SignalInfo={'Force_sensor_1','8','16','BE','unsigned','Standard','0','1','0','-Inf','Inf';'Force_sensor_2','24','16','BE','unsigned','Standard','0','1','0','-Inf','Inf';'Force_sensor_3','40','16','BE','unsigned','Standard','0','1','0','-Inf','Inf';'Force_sensor_4','56','16','BE','unsigned','Standard','0','1','0','-Inf','Inf'}  IDPort=off  TimestampPort=off  ErrorPort=off  RemotePort=off  LengthPort=off  StatusPort=off  ApplyMinMax=off
      settings: DataFormat=CANdb specified signals
  CAN Unpack9 : canmsglib/CAN Unpack  CANdbFile=E:\OneDrive\OneDrive - The Chinese University of Hong Kong\文档\Research\SRIL\12nd\Experiment\Simulink\RoboModule0729.dbc  MsgList=Feedback_curvelpos_Dv1  MsgName=Feedback_curvelpos_Dv1  MsgIDType=Standard (11-bit identifier)  MsgIdentifier=27  MsgLength=8  SignalInfo={'real_current','8','16','BE','signed','Standard','0','1','0','-Inf','Inf';'real_position','56','32','BE','signed','Standard','0','1','0','-Inf','Inf';'real_velocity','24','16','BE','signed','Standard','0','1','0','-Inf','Inf'}  IDPort=off  TimestampPort=off  ErrorPort=off  RemotePort=off  LengthPort=off  StatusPort=off  ApplyMinMax=off
      settings: DataFormat=CANdb specified signals
  Display{1..5,8} (6 alike) : Display
      settings: Format=hex (Stored Integer)
  Mux_4_current1 : Mux  Inputs=9
  Scope : Scope
  Scope1 : Scope
  Scope2 : Scope
  Terminator{8..10,13..14,20,26..27,32,34} (10 alike) : Terminator
  Outport1 : Outport
  wires:
  [Pos_Motor_2] -> Mux_4_current1/2  "Pos_Motor_2"
  [Pos_Motor_3] -> Mux_4_current1/3  "Pos_Motor_3"
  [Pos_Motor_5] -> Mux_4_current1/5  "Pos_Motor_5"
  [Cable_tension_3] -> Mux_4_current1/8  "Cable_tension_3"
  CAN Unpack7/2 -> Display5/1, [Pos_Motor_4]
  [Cable_tension_4] -> Mux_4_current1/9  "Cable_tension_4"
  CAN Unpack9/1 -> Terminator9/1  "motor1_current"
  CAN Unpack8/3 -> Scope1/1, [Cable_tension_3]
  [Cable_tension_1] -> Mux_4_current1/6  "Cable_tension_1"
  CAN Unpack15/3 -> Terminator14/1
  CAN Unpack9/2 -> Display8/1, [Pos_Motor_1]
  CAN Unpack7/3 -> Terminator34/1
  CAN Unpack5/1 -> Terminator26/1
  CAN Unpack6/2 -> Display3/1, [Pos_Motor_3]
  [CANMsg] -> CAN Unpack6/1
  CAN Unpack5/2 -> Display1/1, [Pos_Motor_2]
  [CANMsg] -> CAN Unpack15/1
  CAN Unpack15/2 -> Display2/1, [Pos_Motor_5]
  CAN Unpack6/3 -> Terminator27/1
  CAN Unpack8/2 -> Scope/1, [Cable_tension_2]
  CAN Unpack8/1 -> Display4/1, [Cable_tension_1]
  CAN Unpack9/3 -> Terminator8/1
  CAN Unpack5/3 -> Terminator20/1
  CAN Unpack6/1 -> Terminator32/1
  Mux_4_current1/1 -> Outport1/1
  [CANMsg] -> CAN Unpack5/1
  [CANMsg] -> CAN Unpack7/1
  In2/1 -> CAN Unpack9/1, [CANMsg]
  CAN Unpack15/1 -> Terminator10/1
  [Cable_tension_2] -> Mux_4_current1/7  "Cable_tension_2"
  CAN Unpack8/4 -> Scope2/1, [Cable_tension_4]
  [Pos_Motor_1] -> Mux_4_current1/1  "Pos_Motor_1"
  [CANMsg] -> CAN Unpack8/1
  [Pos_Motor_4] -> Mux_4_current1/4  "Pos_Motor_4"
  CAN Unpack7/1 -> Terminator13/1

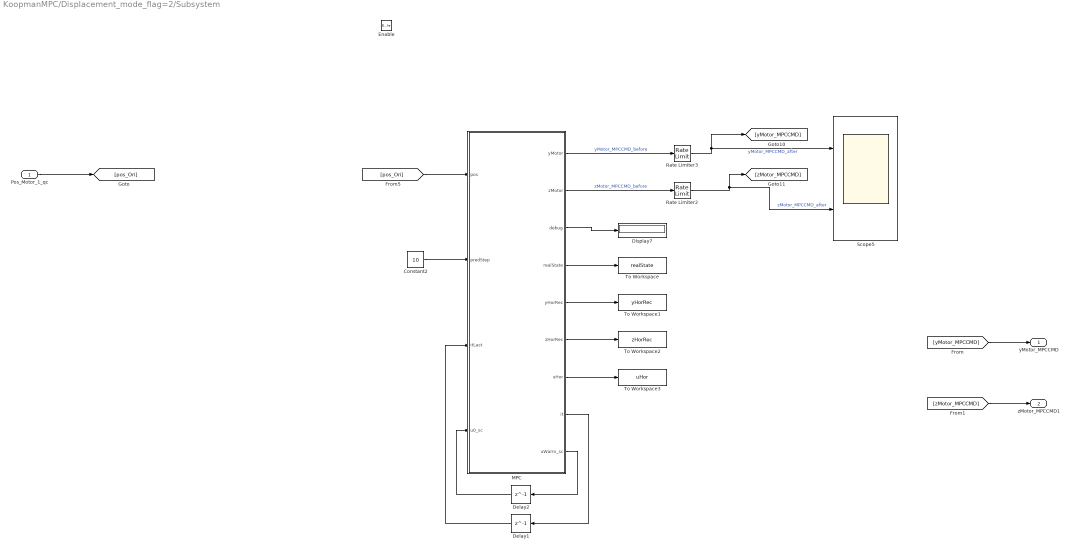
== system KoopmanMPC/Displacement_mode_flag=2/Subsystem ==
  Pos_Motor_1_qc : Inport
  Enable : EnablePort  StatesWhenEnabling=reset
  Constant2 : Constant  Value=10
  Delay1 : Delay  DelayLength=1  InitialCondition=1
  Delay2 : Delay  DelayLength=1  InitialCondition=1*ones(20,1)
  Display7 : Display
  MPC : MATLAB Function  LoadFcn=|  TreatAsAtomicUnit=on
      | clearvars
      | clc
      | load('MtxMPC.mat')
      | load('figure8_final_trajectory.mat')
  Rate Limiter2 : RateLimiter  SampleTimeMode=inherited
  Rate Limiter3 : RateLimiter  SampleTimeMode=inherited
  Scope5 : Scope  NumInputPorts=2
  To Workspace : ToWorkspace  VariableName=realState  SaveFormat=Timeseries  SampleTime=-1
  To Workspace1 : ToWorkspace  VariableName=yHorRec  SaveFormat=Timeseries  SampleTime=-1
  To Workspace2 : ToWorkspace  VariableName=zHorRec  SaveFormat=Timeseries  SampleTime=-1
  To Workspace3 : ToWorkspace  VariableName=uHor  SaveFormat=Timeseries  SampleTime=-1
  yMotor_MPCCMD : Outport
  zMotor_MPCCMD1 : Outport  Port=2
  wires:
  MPC/3(debug) -> Display7/1
  Delay2/1 -> MPC/4(u0_sc)
  MPC/7(uHor) -> To Workspace3/1
  Delay1/1 -> MPC/3(itLast)
  MPC/1(yMotor) -> Rate Limiter3/1  "yMotor_MPCCMD_before"
  [pos_Ori] -> MPC/1(pos)
  Rate Limiter2/1 -> [zMotor_MPCCMD], Scope5/2  "zMotor_MPCCMD_after"
  MPC/8(it) -> Delay1/1
  MPC/4(realState) -> To Workspace/1
  MPC/5(yHorRec) -> To Workspace1/1
  MPC/6(zHorRec) -> To Workspace2/1
  Constant2/1 -> MPC/2(predStep)
  MPC/9(uWarm_sc) -> Delay2/1
  Rate Limiter3/1 -> [yMotor_MPCCMD], Scope5/1  "yMotor_MPCCMD_after"
  MPC/2(zMotor) -> Rate Limiter2/1  "zMotor_MPCCMD_before"
  Pos_Motor_1_qc/1 -> [pos_Ori]
  [zMotor_MPCCMD] -> zMotor_MPCCMD1/1
  [yMotor_MPCCMD] -> yMotor_MPCCMD/1

== system KoopmanMPC/Displacement_mode_flag=2/Subsystem1 ==
  position_in : Inport
  Enable : EnablePort
  position_out : Outport
  wires:
  position_in/1 -> position_out/1

== system KoopmanMPC/Displacement_mode_flag=2/Subsystem2 ==
  position_in : Inport
  Enable : EnablePort
  position_out : Outport
  wires:
  position_in/1 -> position_out/1

== system KoopmanMPC/Displacement_mode_flag=2/Subsystem3 ==
  position_in : Inport
  Enable : EnablePort
  position_out : Outport
  wires:
  position_in/1 -> position_out/1

== system KoopmanMPC/Displacement_mode_flag=2/Subsystem5 ==
  position_in : Inport
  Enable : EnablePort
  position_out : Outport
  wires:
  position_in/1 -> position_out/1

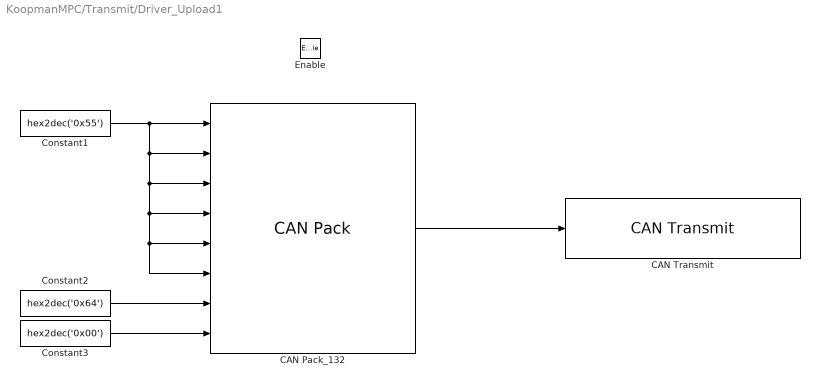
== system KoopmanMPC/Transmit/Driver_Upload1 ==
  Enable : EnablePort  StatesWhenEnabling=reset
  CAN Pack_132 : canmsglib/CAN Pack  CANdbFile=E:\Research\SRIL\9th\Mnp_Control_Sim\RoboModule0611.dbc  MsgList=Configuration_all  MsgName=Configuration_all  MsgIDType=Standard (11-bit identifier)  MsgIdentifier=10  MsgLength=8  Remote=off  ApplyMinMax=off  BusOutput=off  SignalInfo={'Data2','16','8','BE','unsigned','Standard','0','1','0','-Inf','Inf';'Data3','24','8','BE','unsigned','Standard','0','1','0','-Inf','Inf';'Data4','32','8','BE','unsigned','Standard','0','1','0','-Inf','Inf';'Data5','40','8','BE','unsigned','Standard','0','1','0','-Inf','Inf';'Data6','48','8','BE','unsigned','Standard','0','1','0','-Inf','Inf';'Data7','56','8','BE','unsigned','Standard','0','1','0','-Inf','Inf';'output_cycle_curvelpos','0','8','BE','unsigned','Standard','0','1','0','-Inf','Inf';'output_cycle_others','8','8','BE','unsigned','Standard','0','1','0','-Inf','Inf'}
      settings: DataFormat=CANdb specified signals
  CAN Transmit : canlib/CAN Transmit  BlockHandle=7808.0001  Device=PEAK-System PCAN-USB (PCAN_USBBUS1)  DeviceMenu=PEAK-System PCAN-USB (PCAN_USBBUS1)  ObjConstructor=canChannel('PEAK-System', 'PCAN_USBBUS1')  EnableEventTransmit=off  EnablePeriodicTransmit=off  MessagePeriod=1.000
  Constant1 : Constant  Value=hex2dec('0x55')  OutDataTypeStr=uint8  SampleTime=-1
  Constant2 : Constant  Value=hex2dec('0x64')  OutDataTypeStr=uint8  SampleTime=-1
  Constant3 : Constant  Value=hex2dec('0x00')  OutDataTypeStr=uint8  SampleTime=-1
  wires:
  Constant1/1 -> CAN Pack_132/3, CAN Pack_132/5, CAN Pack_132/6, CAN Pack_132/4, CAN Pack_132/2, CAN Pack_132/1
  CAN Pack_132/1 -> CAN Transmit/1
  Constant2/1 -> CAN Pack_132/7
  Constant3/1 -> CAN Pack_132/8

== system KoopmanMPC/Transmit/Mode Selection1 ==
  Enable : EnablePort  StatesWhenEnabling=reset
  CAN Pack_132 : canmsglib/CAN Pack  CANdbFile=E:\Research\SRIL\7th\28379Project\Laser_Manipulator_Control\RoboModule.dbc  MsgList=(none)  MsgName=Mode_Selection  MsgIDType=Standard (11-bit identifier)  MsgIdentifier=1  MsgLength=8  Remote=off  ApplyMinMax=off  BusOutput=off  SignalInfo={'Data1','8','8','BE','unsigned','Standard','0','1','0','-Inf','Inf';'Data2','16','8','BE','unsigned','Standard','0','1','0','-Inf','Inf';'Data3','24','8','BE','unsigned','Standard','0','1','0','-Inf','Inf';'Data4','32','8','BE','unsigned','Standard','0','1','0','-Inf','Inf';'Data5','40','8','BE','unsigned','Standard','0','1','0','-Inf','Inf';'Data6','48','8','BE','unsigned','Standard','0','1','0','-Inf','Inf';'Data7','56','8','BE','unsigned','Standard','0','1','0','-Inf','Inf';'Mode','0','8','BE','unsigned','Standard','0','1','0','-Inf','Inf'}
      settings: DataFormat=CANdb specified signals
  CAN Transmit : canlib/CAN Transmit  BlockHandle=7851.0001  Device=PEAK-System PCAN-USB (PCAN_USBBUS1)  DeviceMenu=PEAK-System PCAN-USB (PCAN_USBBUS1)  ObjConstructor=canChannel('PEAK-System', 'PCAN_USBBUS1')  EnableEventTransmit=off  EnablePeriodicTransmit=off  MessagePeriod=1.000
  Constant1 : Constant  Value=hex2dec('0x55')  OutDataTypeStr=uint8  SampleTime=-1
  Mode Number : Constant  Value=hex2dec('0x04')  OutDataTypeStr=uint8  SampleTime=-1
  wires:
  CAN Pack_132/1 -> CAN Transmit/1
  Constant1/1 -> CAN Pack_132/7, CAN Pack_132/6, CAN Pack_132/5, CAN Pack_132/4, CAN Pack_132/3, CAN Pack_132/2, CAN Pack_132/1
  Mode Number/1 -> CAN Pack_132/8

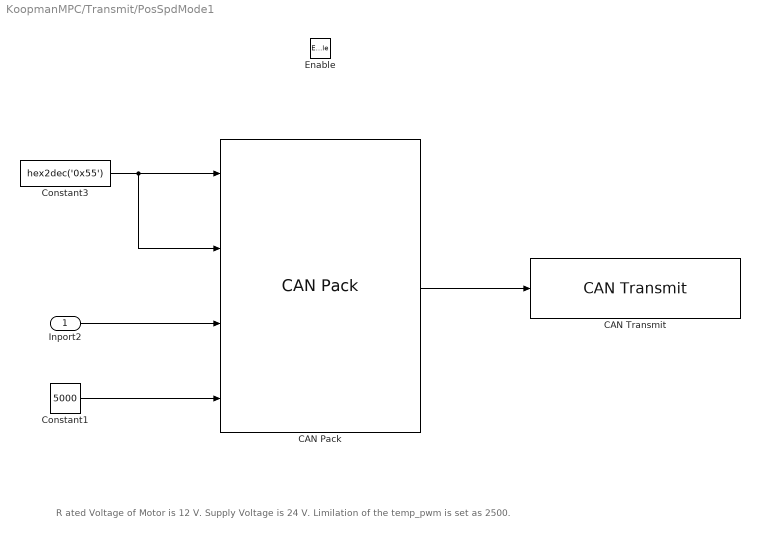
== system KoopmanMPC/Transmit/PosSpdMode1 ==
  note: R ated Voltage of Motor is 12 V. Supply Voltage is 24 V. Limilation of the temp_pwm is set as 2500.
  Inport2 : Inport
  Enable : EnablePort
  CAN Pack : canmsglib/CAN Pack  CANdbFile=E:\OneDrive\OneDrive - The Chinese University of Hong Kong\文档\Research\SRIL\12nd\Experiment\Simulink\RoboModule0729.dbc  MsgList=Position_Dr1  MsgName=Position_Dr1  MsgIDType=Standard (11-bit identifier)  MsgIdentifier=21  MsgLength=8  Remote=off  ApplyMinMax=off  BusOutput=off  SignalInfo={'Data2','16','8','BE','unsigned','Standard','0','1','0','-Inf','Inf';'Data3','24','8','BE','unsigned','Standard','0','1','0','-Inf','Inf';'temp_position','56','32','BE','signed','Standard','0','1','0','-Inf','Inf';'temp_pwm','8','16','BE','unsigned','Standard','0','1','0','-Inf','Inf'}
      settings: DataFormat=CANdb specified signals
  CAN Transmit : canlib/CAN Transmit  BlockHandle=7874.0001  Device=PEAK-System PCAN-USB (PCAN_USBBUS1)  DeviceMenu=PEAK-System PCAN-USB (PCAN_USBBUS1)  ObjConstructor=canChannel('PEAK-System', 'PCAN_USBBUS1')  EnableEventTransmit=off  EnablePeriodicTransmit=on  MessagePeriod=0.01
  Constant1 : Constant  Value=5000
  Constant3 : Constant  Value=hex2dec('0x55')  OutDataTypeStr=uint8  SampleTime=-1
  wires:
  Constant3/1 -> CAN Pack/2, CAN Pack/1
  Inport2/1 -> CAN Pack/3
  Constant1/1 -> CAN Pack/4
  CAN Pack/1 -> CAN Transmit/1

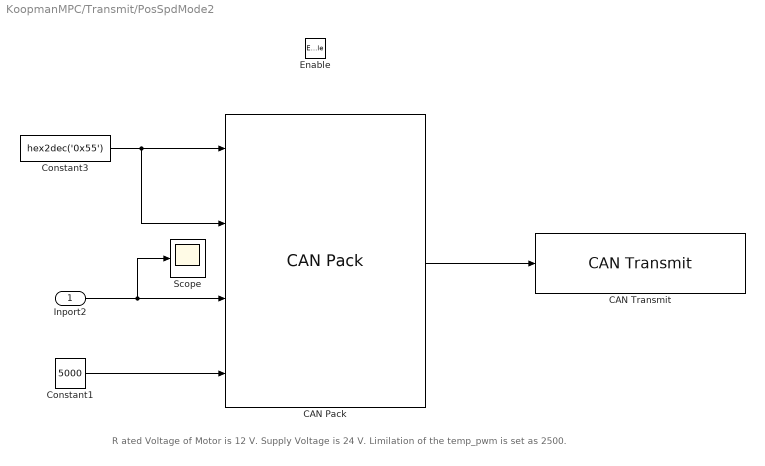
== system KoopmanMPC/Transmit/PosSpdMode2 ==
  note: R ated Voltage of Motor is 12 V. Supply Voltage is 24 V. Limilation of the temp_pwm is set as 2500.
  Inport2 : Inport
  Enable : EnablePort
  CAN Pack : canmsglib/CAN Pack  CANdbFile=E:\Research\SRIL\12nd\Simulink\RoboModule0729.dbc  MsgList=Position_Dr2  MsgName=Position_Dr2  MsgIDType=Standard (11-bit identifier)  MsgIdentifier=37  MsgLength=8  Remote=off  ApplyMinMax=off  BusOutput=off  SignalInfo={'Data2','16','8','BE','unsigned','Standard','0','1','0','-Inf','Inf';'Data3','24','8','BE','unsigned','Standard','0','1','0','-Inf','Inf';'temp_position','56','32','BE','signed','Standard','0','1','0','-Inf','Inf';'temp_pwm','8','16','BE','unsigned','Standard','0','1','0','-Inf','Inf'}
      settings: DataFormat=CANdb specified signals
  CAN Transmit : canlib/CAN Transmit  BlockHandle=7888.0001  Device=PEAK-System PCAN-USB (PCAN_USBBUS1)  DeviceMenu=PEAK-System PCAN-USB (PCAN_USBBUS1)  ObjConstructor=canChannel('PEAK-System', 'PCAN_USBBUS1')  EnableEventTransmit=off  EnablePeriodicTransmit=on  MessagePeriod=0.01
  Constant1 : Constant  Value=5000
  Constant3 : Constant  Value=hex2dec('0x55')  OutDataTypeStr=uint8  SampleTime=-1
  Scope : Scope
  wires:
  CAN Pack/1 -> CAN Transmit/1
  Constant3/1 -> CAN Pack/2, CAN Pack/1
  Inport2/1 -> Scope/1, CAN Pack/3
  Constant1/1 -> CAN Pack/4

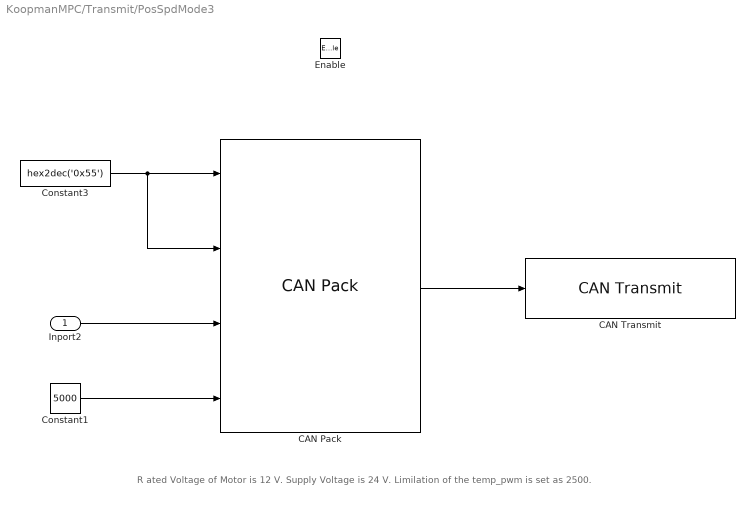
== system KoopmanMPC/Transmit/PosSpdMode3 ==
  note: R ated Voltage of Motor is 12 V. Supply Voltage is 24 V. Limilation of the temp_pwm is set as 2500.
  Inport2 : Inport
  Enable : EnablePort
  CAN Pack : canmsglib/CAN Pack  CANdbFile=E:\OneDrive\OneDrive - The Chinese University of Hong Kong\文档\Research\SRIL\12nd\Experiment\Simulink\RoboModule0729.dbc  MsgList=Position_Dr3  MsgName=Position_Dr3  MsgIDType=Standard (11-bit identifier)  MsgIdentifier=53  MsgLength=8  Remote=off  ApplyMinMax=off  BusOutput=off  SignalInfo={'Data2','16','8','BE','unsigned','Standard','0','1','0','-Inf','Inf';'Data3','24','8','BE','unsigned','Standard','0','1','0','-Inf','Inf';'temp_position','56','32','BE','signed','Standard','0','1','0','-Inf','Inf';'temp_pwm','8','16','BE','unsigned','Standard','0','1','0','-Inf','Inf'}
      settings: DataFormat=CANdb specified signals
  CAN Transmit : canlib/CAN Transmit  BlockHandle=7905.0001  Device=PEAK-System PCAN-USB (PCAN_USBBUS1)  DeviceMenu=PEAK-System PCAN-USB (PCAN_USBBUS1)  ObjConstructor=canChannel('PEAK-System', 'PCAN_USBBUS1')  EnableEventTransmit=off  EnablePeriodicTransmit=on  MessagePeriod=0.01
  Constant1 : Constant  Value=5000
  Constant3 : Constant  Value=hex2dec('0x55')  OutDataTypeStr=uint8  SampleTime=-1
  wires:
  CAN Pack/1 -> CAN Transmit/1
  Constant3/1 -> CAN Pack/2, CAN Pack/1
  Inport2/1 -> CAN Pack/3
  Constant1/1 -> CAN Pack/4

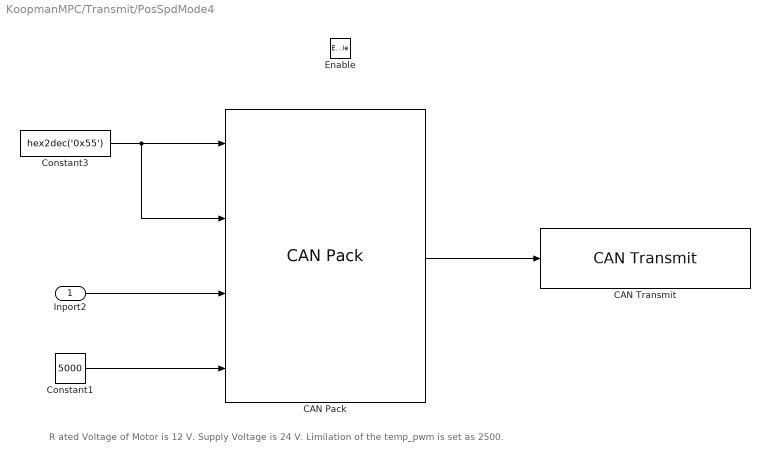
== system KoopmanMPC/Transmit/PosSpdMode4 ==
  note: R ated Voltage of Motor is 12 V. Supply Voltage is 24 V. Limilation of the temp_pwm is set as 2500.
  Inport2 : Inport
  Enable : EnablePort
  CAN Pack : canmsglib/CAN Pack  CANdbFile=E:\OneDrive\OneDrive - The Chinese University of Hong Kong\文档\Research\SRIL\12nd\Experiment\Simulink\RoboModule0729.dbc  MsgList=Position_Dr4  MsgName=Position_Dr4  MsgIDType=Standard (11-bit identifier)  MsgIdentifier=69  MsgLength=8  Remote=off  ApplyMinMax=off  BusOutput=off  SignalInfo={'Data2','16','8','BE','unsigned','Standard','0','1','0','-Inf','Inf';'Data3','24','8','BE','unsigned','Standard','0','1','0','-Inf','Inf';'temp_position','56','32','BE','signed','Standard','0','1','0','-Inf','Inf';'temp_pwm','8','16','BE','unsigned','Standard','0','1','0','-Inf','Inf'}
      settings: DataFormat=CANdb specified signals
  CAN Transmit : canlib/CAN Transmit  BlockHandle=7919.0001  Device=PEAK-System PCAN-USB (PCAN_USBBUS1)  DeviceMenu=PEAK-System PCAN-USB (PCAN_USBBUS1)  ObjConstructor=canChannel('PEAK-System', 'PCAN_USBBUS1')  EnableEventTransmit=off  EnablePeriodicTransmit=on  MessagePeriod=0.01
  Constant1 : Constant  Value=5000
  Constant3 : Constant  Value=hex2dec('0x55')  OutDataTypeStr=uint8  SampleTime=-1
  wires:
  CAN Pack/1 -> CAN Transmit/1
  Constant3/1 -> CAN Pack/2, CAN Pack/1
  Inport2/1 -> CAN Pack/3
  Constant1/1 -> CAN Pack/4

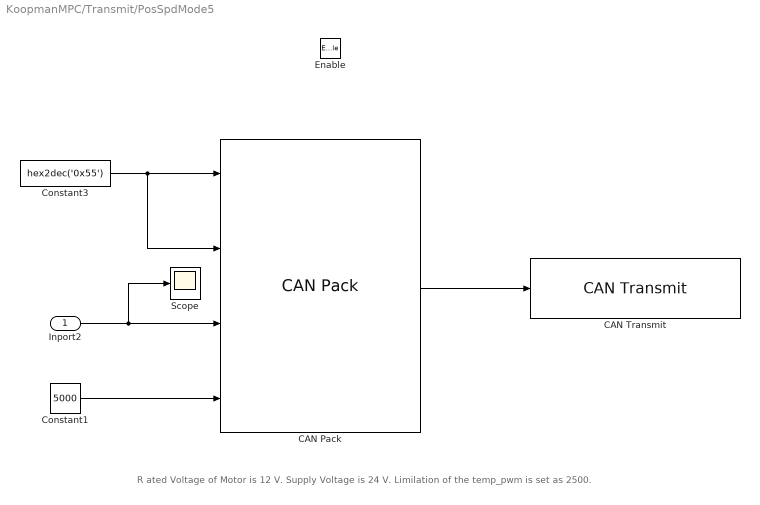
== system KoopmanMPC/Transmit/PosSpdMode5 ==
  note: R ated Voltage of Motor is 12 V. Supply Voltage is 24 V. Limilation of the temp_pwm is set as 2500.
  Inport2 : Inport
  Enable : EnablePort
  CAN Pack : canmsglib/CAN Pack  CANdbFile=E:\OneDrive\OneDrive - The Chinese University of Hong Kong\文档\Research\SRIL\12nd\Experiment\Simulink\RoboModule0729.dbc  MsgList=Position_Dr5  MsgName=Position_Dr5  MsgIDType=Standard (11-bit identifier)  MsgIdentifier=85  MsgLength=8  Remote=off  ApplyMinMax=off  BusOutput=off  SignalInfo={'Data2','16','8','BE','unsigned','Standard','0','1','0','-Inf','Inf';'Data3','24','8','BE','unsigned','Standard','0','1','0','-Inf','Inf';'temp_position','56','32','BE','signed','Standard','0','1','0','-Inf','Inf';'temp_pwm','8','16','BE','unsigned','Standard','0','1','0','-Inf','Inf'}
      settings: DataFormat=CANdb specified signals
  CAN Transmit : canlib/CAN Transmit  BlockHandle=7933.0001  Device=PEAK-System PCAN-USB (PCAN_USBBUS1)  DeviceMenu=PEAK-System PCAN-USB (PCAN_USBBUS1)  ObjConstructor=canChannel('PEAK-System', 'PCAN_USBBUS1')  EnableEventTransmit=off  EnablePeriodicTransmit=on  MessagePeriod=0.01
  Constant1 : Constant  Value=5000
  Constant3 : Constant  Value=hex2dec('0x55')  OutDataTypeStr=uint8  SampleTime=-1
  Scope : Scope
  wires:
  CAN Pack/1 -> CAN Transmit/1
  Constant3/1 -> CAN Pack/2, CAN Pack/1
  Inport2/1 -> Scope/1, CAN Pack/3
  Constant1/1 -> CAN Pack/4

== system KoopmanMPC/Transmit/Reset ==
  Enable : EnablePort  StatesWhenEnabling=reset
  CAN Pack_132 : canmsglib/CAN Pack  CANdbFile=E:\Research\SRIL\7th\28379Project\Laser_Manipulator_Control\RoboModule.dbc  MsgList=(none)  MsgName=Reset  MsgIDType=Standard (11-bit identifier)  MsgIdentifier=0  MsgLength=8  Remote=off  ApplyMinMax=off  BusOutput=off  SignalInfo={'Data0','0','8','BE','unsigned','Standard','0','1','0','-Inf','Inf';'Data1','8','8','BE','unsigned','Standard','0','1','0','-Inf','Inf';'Data2','16','8','BE','unsigned','Standard','0','1','0','-Inf','Inf';'Data3','24','8','BE','unsigned','Standard','0','1','0','-Inf','Inf';'Data4','32','8','BE','unsigned','Standard','0','1','0','-Inf','Inf';'Data5','40','8','BE','unsigned','Standard','0','1','0','-Inf','Inf';'Data6','48','8','BE','unsigned','Standard','0','1','0','-Inf','Inf';'Data7','56','8','BE','unsigned','Standard','0','1','0','-Inf','Inf'}
      settings: DataFormat=CANdb specified signals
  CAN Transmit : canlib/CAN Transmit  BlockHandle=7950.0001  Device=PEAK-System PCAN-USB (PCAN_USBBUS1)  DeviceMenu=PEAK-System PCAN-USB (PCAN_USBBUS1)  ObjConstructor=canChannel('PEAK-System', 'PCAN_USBBUS1')  EnableEventTransmit=off  EnablePeriodicTransmit=off  MessagePeriod=1.000
  Constant1 : Constant  Value=hex2dec('0x55')  OutDataTypeStr=uint8  SampleTime=-1
  wires:
  Constant1/1 -> CAN Pack_132/3, CAN Pack_132/5, CAN Pack_132/6, CAN Pack_132/7, CAN Pack_132/8, CAN Pack_132/4, CAN Pack_132/2, CAN Pack_132/1
  CAN Pack_132/1 -> CAN Transmit/1

== system KoopmanMPC/Transmit/Reset_Manually ==
  Enable : EnablePort  StatesWhenEnabling=reset
  Trigger : TriggerPort  VariantControl=(inherit)  PortDimensions=1
  CAN Pack : canmsglib/CAN Pack  CANdbFile=E:\OneDrive\OneDrive - The Chinese University of Hong Kong\文档\Research\SRIL\12nd\Experiment\Simulink\RoboModule0729.dbc  MsgList=Reset_all  MsgName=Reset_all  MsgIDType=Standard (11-bit identifier)  MsgIdentifier=0  MsgLength=8  Remote=off  ApplyMinMax=off  BusOutput=off  SignalInfo={'Data0','0','8','BE','unsigned','Standard','0','1','0','-Inf','Inf';'Data1','8','8','BE','unsigned','Standard','0','1','0','-Inf','Inf';'Data2','16','8','BE','unsigned','Standard','0','1','0','-Inf','Inf';'Data3','24','8','BE','unsigned','Standard','0','1','0','-Inf','Inf';'Data4','32','8','BE','unsigned','Standard','0','1','0','-Inf','Inf';'Data5','40','8','BE','unsigned','Standard','0','1','0','-Inf','Inf';'Data6','48','8','BE','unsigned','Standard','0','1','0','-Inf','Inf';'Data7','56','8','BE','unsigned','Standard','0','1','0','-Inf','Inf'}
      settings: DataFormat=CANdb specified signals
  CAN Transmit : canlib/CAN Transmit  BlockHandle=7972.0001  Device=PEAK-System PCAN-USB (PCAN_USBBUS1)  DeviceMenu=PEAK-System PCAN-USB (PCAN_USBBUS1)  ObjConstructor=canChannel('PEAK-System', 'PCAN_USBBUS1')  EnableEventTransmit=off  EnablePeriodicTransmit=on  MessagePeriod=0.01
  Constant2 : Constant  Value=hex2dec('0x55')  OutDataTypeStr=uint8  SampleTime=-1
  wires:
  CAN Pack/1 -> CAN Transmit/1
  Constant2/1 -> CAN Pack/1, CAN Pack/3, CAN Pack/5, CAN Pack/6, CAN Pack/7, CAN Pack/8, CAN Pack/4, CAN Pack/2

== matlab function KoopmanMPC/Displacement_mode_flag=2/MATLAB Function2 ==
  data: pos_x input; Pos_rel output; pos_y input; it output; pos_z input; itLast input; enableLast input; enable output
function [Pos_rel,it,enable] = allocation(pos_x,pos_y,pos_z,itLast,enableLast)
Pos_now = [pos_x,pos_y,pos_z];

Pos0 = [18.54,78.56,-119.465];


Pos_rel = Pos_now - Pos0;

if enableLast ~= 1
    if abs(Pos_rel(2) - 4) < 0.3 && abs(Pos_rel(3) - (-2)) < 0.3
        enable = 1;
    else
        enable = enableLast;
    end
else
    enable = enableLast;
end

it = itLast + 1;
end

== matlab function KoopmanMPC/Initial_flag=1/RandomControlSequence ==
  settings: updateMethod=DISCRETE
  data: u output; force_meas input; F_min input; F_max input; step input
function u = tension_control(force_meas,F_min,F_max,step)
    u_pull = step; % small constant torque or velocity
    u_relax = -step;
    
    if force_meas < F_min
        u = u_pull;
    elseif force_meas > F_max
        u = u_relax;
    else
        u = 0; % hold
    end
end

== matlab function KoopmanMPC/Initial_flag=1/RandomControlSequence1 ==
  settings: updateMethod=DISCRETE
  data: u output; force_meas input; F_min input; F_max input; step input
function u = tension_control(force_meas,F_min,F_max,step)
    u_pull = step; % small constant torque or velocity
    u_relax = -step;
    
    if force_meas < F_min
        u = u_pull;
    elseif force_meas > F_max
        u = u_relax;
    else
        u = 0; % hold
    end
end

== matlab function KoopmanMPC/Initial_flag=1/RandomControlSequence2 ==
  settings: updateMethod=DISCRETE
  data: u output; force_meas input; F_min input; F_max input; step input
function u = tension_control(force_meas,F_min,F_max,step)
    u_pull = step; % small constant torque or velocity
    u_relax = -step;
    
    if force_meas < F_min
        u = u_pull;
    elseif force_meas > F_max
        u = u_relax;
    else
        u = 0; % hold
    end
end
